simulink model "caracciolo"  (R2023b)
settings: Solver=FixedStepAuto  StartTime=0.0  StopTime=50  FixedStep=0.05  RelTol=1e-3
values from neighbouring files (symbols this model uses):
  a = 0.8    [init.m]
  b = 0.8    [init.m]
  d0 = 0.5    [init.m]
  fr = 0.005    [init.m]
  g = -9.8    [init.m]
  m = 550    [init.m]
  M = diag([m; m; I])    [init.m]
  M_inv = inv(M)    [init.m]
  mu = 0.9    [init.m]
  r = 0.3    [init.m]
  state0 = [0; 0; 0.2]    [init.m]
  tau_max = 3.88*2    (= 7.76)    [init.m]
  tau_min = -tau_max    (= -7.76)    [init.m]
libraries: simulink x1
settings Model: Creator=agisi2  LastModifiedBy=agisi2

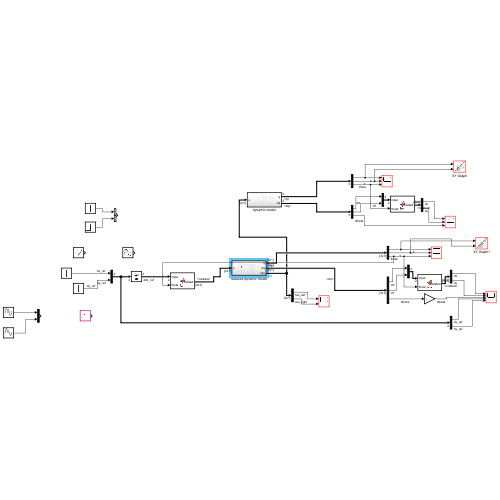
[thumbnail: Simulink's stored preview of the top-level diagram]
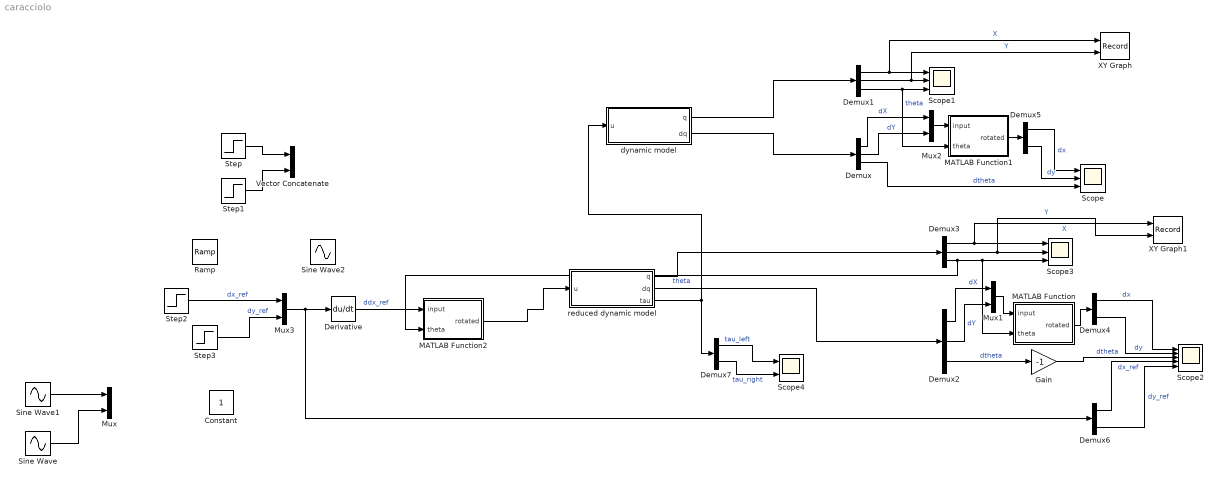
== system caracciolo ==
  Constant : Constant
  Demux{,1..3} (4 alike) : Demux  Outputs=3
  Demux{4..7} (4 alike) : Demux  Outputs=2
  Derivative : Derivative
  Gain : Gain  Gain=-1
  MATLAB Function : MATLAB Function  TreatAsAtomicUnit=on
  MATLAB Function1 : MATLAB Function  TreatAsAtomicUnit=on
  MATLAB Function2 : MATLAB Function  TreatAsAtomicUnit=on
  Mux{,1..3} (4 alike) : Mux  Inputs=2
  Ramp : simulink/Sources/Ramp  slope=1  start=1  InitialOutput=0
  Scope : Scope  NumInputPorts=3
  Scope1 : Scope  NumInputPorts=3
  Scope2 : Scope  NumInputPorts=5
  Scope3 : Scope  NumInputPorts=3
  Scope4 : Scope  NumInputPorts=2
  Sine Wave : Sin  SampleTime=0
  Sine Wave1 : Sin  SampleTime=0
  Sine Wave2 : Sin  SampleTime=0
  Step : Step  After=-2  SampleTime=0
  Step1 : Step  SampleTime=0
  Step2 : Step  Time=0.1  SampleTime=0
  Step3 : Step  Time=0.1  After=0  SampleTime=0
  Vector Concatenate : Concatenate
  XY Graph : Record  FileSettingsInternal="{\"entries\":[{\"content\":{\"excelSettings\":{\"content\":{},\"type\":\"Streamout.ExcelSettings\"}},\"type\":\"Streamout.FileSettingStorage\",\"uuid\":\"\"}],\"packageUris\":[\"http:\\/\\/schema.mathworks.com\\/mf0\\/streamout_blocks\\/R2020a\"],\"version\":\"1.0\"}"  Layout=[2 1]  SignalsInternal="{\"entries\":[{\"content\":{\"signals\":[{\"content\":{\"blockPath\":[],\"dimensions\":[1],\"domain\":\"\",\"lineColor\":\"#a2142f\",\"plots\":[1],\"port\":1,\"sid\":[\"\"],\"signalID\":5305,\"signalName\":\"X\"},\"type\":\"RecordBlkView.Signal\",\"uuid\":\"\"},{\"content\":{\"blockPath\":[],\"dimensions\":[1],\"domain\":\"\",\"lineColor\":\"#139fff\",\"plots\":[1],\"port\":2,\"sid\":[\"\"],\"signalID\":5309,\"signalName\":\"Y\"},\"type\":\"RecordBlkView.Signal\",\"uuid\":\"\"}]},\"type\":\"RecordBlkView.InputSignals\",\"uuid\":\"\"}],\"packageUris\":[\"http:\\/\\/schema.mathworks.com\\/mf0\\/streamout_blocks\\/R2020a\"],\"version\":\"1.0\"}"  VisualizationBindings="{\"xyplotplugin\":{\"info\":[{\"series\":[{\"bindingParametersList\":[{\"parameter\":\"X-Axis\",\"signalID\":5305,\"signalName\":\"X\"},{\"parameter\":\"Y-Axis\",\"signalID\":5309,\"signalName\":\"Y\"}],\"seriesID\":39005}],\"subplotID\":1},{\"series\":[],\"subplotID\":2}]}}"  CompatibilityTag=XY
  XY Graph1 : Record  FileSettingsInternal="{\"entries\":[{\"content\":{\"excelSettings\":{\"content\":{},\"type\":\"Streamout.ExcelSettings\"}},\"type\":\"Streamout.FileSettingStorage\",\"uuid\":\"\"}],\"packageUris\":[\"http:\\/\\/schema.mathworks.com\\/mf0\\/streamout_blocks\\/R2020a\"],\"version\":\"1.0\"}"  Layout=[1 1]  SignalsInternal="{\"entries\":[{\"content\":{\"signals\":[{\"content\":{\"blockPath\":[],\"dimensions\":[1,1],\"domain\":\"\",\"lineColor\":\"#a2142f\",\"plots\":[1],\"port\":1,\"sid\":[\"\"],\"signalID\":5313,\"signalName\":\"X\"},\"type\":\"RecordBlkView.Signal\",\"uuid\":\"\"},{\"content\":{\"blockPath\":[],\"dimensions\":[1,1],\"domain\":\"\",\"lineColor\":\"#139fff\",\"plots\":[1],\"port\":2,\"sid\":[\"\"],\"signalID\":5317,\"signalName\":\"Y\"},\"type\":\"RecordBlkView.Signal\",\"uuid\":\"\"}]},\"type\":\"RecordBlkView.InputSignals\",\"uuid\":\"\"}],\"packageUris\":[\"http:\\/\\/schema.mathworks.com\\/mf0\\/streamout_blocks\\/R2020a\"],\"version\":\"1.0\"}"  VisualizationBindings="{\"xyplotplugin\":{\"info\":[{\"series\":[{\"bindingParametersList\":[{\"parameter\":\"X-Axis\",\"signalID\":5313,\"signalName\":\"X\"},{\"parameter\":\"Y-Axis\",\"signalID\":5317,\"signalName\":\"Y\"}],\"seriesID\":47435}],\"subplotID\":1}]}}"  CompatibilityTag=XY
  dynamic model : Subsystem
  reduced dynamic model : Subsystem
  wires:
  dynamic model/2(dq) -> Demux/1
  dynamic model/1(q) -> Demux1/1
  Demux1/1 -> XY Graph/1, Scope1/1  "X"
  Demux1/2 -> XY Graph/2, Scope1/2  "Y"
  Demux1/3 -> MATLAB Function1/2(theta), Scope1/3  "theta"
  Demux/1 -> Mux2/1  "dX"
  Demux/2 -> Mux2/2  "dY"
  Demux/3 -> Scope/3  "dtheta"
  reduced dynamic model/2(dq) -> Demux2/1
  Demux2/3 -> Gain/1  "dtheta"
  Demux3/1 -> XY Graph1/1, Scope3/1  "X"
  reduced dynamic model/1(q) -> Demux3/1
  Demux3/2 -> XY Graph1/2, Scope3/2  "Y"
  Sine Wave/1 -> Mux/2
  Sine Wave1/1 -> Mux/1
  Step/1 -> Vector Concatenate/1
  Step1/1 -> Vector Concatenate/2
  Demux3/3 -> MATLAB Function2/2(theta), MATLAB Function/2(theta), Scope3/3  "theta"
  Mux1/1 -> MATLAB Function/1(input)
  Demux2/2 -> Mux1/2  "dY"
  Demux2/1 -> Mux1/1  "dX"
  MATLAB Function/1(rotated) -> Demux4/1
  Demux4/1 -> Scope2/1  "dx"
  Demux4/2 -> Scope2/2  "dy"
  Mux2/1 -> MATLAB Function1/1(input)
  MATLAB Function1/1(rotated) -> Demux5/1
  Demux5/1 -> Scope/1  "dx"
  Demux5/2 -> Scope/2  "dy"
  Step3/1 -> Mux3/2  "dy_ref"
  MATLAB Function2/1(rotated) -> reduced dynamic model/1(u)
  Mux3/1 -> Demux6/1, Derivative/1
  Demux6/1 -> Scope2/4  "dx_ref"
  Demux6/2 -> Scope2/5  "dy_ref"
  Step2/1 -> Mux3/1  "dx_ref"
  Derivative/1 -> MATLAB Function2/1(input)  "ddx_ref"
  Gain/1 -> Scope2/3  "dtheta"
  Demux7/1 -> Scope4/1  "tau_left"
  Demux7/2 -> Scope4/2  "tau_right"
  reduced dynamic model/3(tau) -> Demux7/1, dynamic model/1(u)

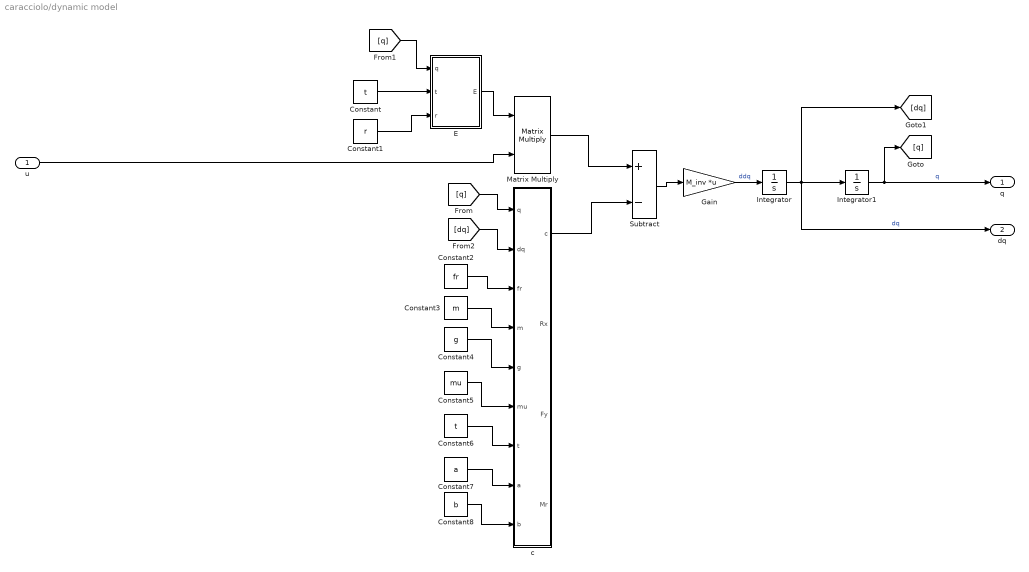
== system caracciolo/dynamic model ==
  u : Inport
  Constant : Constant  Value=t
  Constant1 : Constant  Value=r
  Constant2 : Constant  Value=fr
  Constant3 : Constant  Value=m
  Constant4 : Constant  Value=g
  Constant5 : Constant  Value=mu
  Constant6 : Constant  Value=t
  Constant7 : Constant  Value=a
  Constant8 : Constant  Value=b
  E : MATLAB Function  TreatAsAtomicUnit=on
  Gain : Gain  Gain=M_inv  Multiplication=Matrix(K*u) (u vector)
  Integrator : Integrator
  Integrator1 : Integrator  InitialCondition=state0
  Matrix Multiply : Product  Multiplication=Matrix(*)
  Subtract : Sum  Inputs=+-
  c : MATLAB Function  TreatAsAtomicUnit=on
  q : Outport
  dq : Outport  Port=2
  wires:
  E/1(E) -> Matrix Multiply/1
  u/1 -> Matrix Multiply/2
  Matrix Multiply/1 -> Subtract/1
  c/1(c) -> Subtract/2
  Subtract/1 -> Gain/1
  Gain/1 -> Integrator/1  "ddq"
  Integrator/1 -> dq/1, [dq], Integrator1/1  "dq"
  Integrator1/1 -> q/1, [q]  "q"
  [q] -> c/1(q)
  [q] -> E/1(q)
  [dq] -> c/2(dq)
  Constant/1 -> E/2(t)
  Constant1/1 -> E/3(r)
  Constant2/1 -> c/3(fr)
  Constant3/1 -> c/4(m)
  Constant4/1 -> c/5(g)
  Constant5/1 -> c/6(mu)
  Constant6/1 -> c/7(t)
  Constant7/1 -> c/8(a)
  Constant8/1 -> c/9(b)

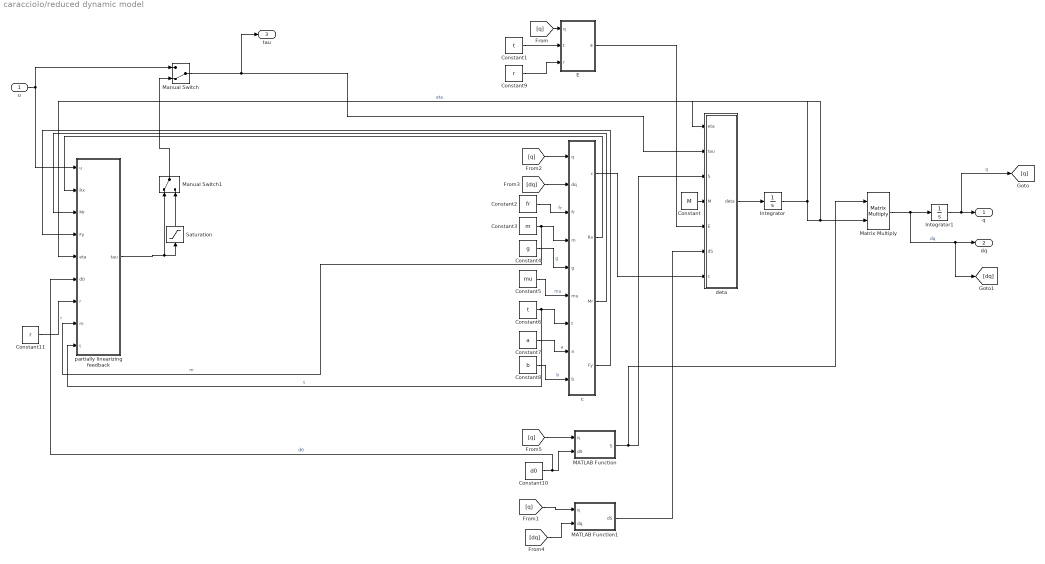
== system caracciolo/reduced dynamic model ==
  u : Inport
  Constant : Constant  Value=M
  Constant1 : Constant  Value=t
  Constant10 : Constant  Value=d0
  Constant11 : Constant  Value=r
  Constant2 : Constant  Value=fr
  Constant3 : Constant  Value=m
  Constant4 : Constant  Value=g
  Constant5 : Constant  Value=mu
  Constant6 : Constant  Value=t
  Constant7 : Constant  Value=a
  Constant8 : Constant  Value=b
  Constant9 : Constant  Value=r
  E : MATLAB Function  TreatAsAtomicUnit=on
  Integrator : Integrator
  Integrator1 : Integrator  InitialCondition=state0
  MATLAB Function : MATLAB Function  TreatAsAtomicUnit=on
  MATLAB Function1 : MATLAB Function  TreatAsAtomicUnit=on
  Manual Switch : ManualSwitch  CurrentSetting=0
  Manual Switch1 : ManualSwitch
  Matrix Multiply : Product  Multiplication=Matrix(*)
  Saturation : Saturate  UpperLimit=tau_max  LowerLimit=tau_min
  c : MATLAB Function  TreatAsAtomicUnit=on
  deta : MATLAB Function  TreatAsAtomicUnit=on
  partially linearizing feedback : MATLAB Function  TreatAsAtomicUnit=on
  q : Outport
  dq : Outport  Port=2
  tau : Outport  Port=3
  wires:
  Constant8/1 -> c/9(b)  "b"
  c/1(c) -> deta/7(c)
  Constant6/1 -> c/7(t), partially linearizing feedback/9(t)  "t"
  Constant4/1 -> c/5(g)  "g"
  Constant3/1 -> c/4(m), partially linearizing feedback/8(m)  "m"
  Constant7/1 -> c/8(a)  "a"
  Constant5/1 -> c/6(mu)  "mu"
  Constant2/1 -> c/3(fr)  "fr"
  Constant1/1 -> E/2(t)
  E/1(E) -> deta/5(E)
  Constant9/1 -> E/3(r)
  MATLAB Function/1(S) -> Matrix Multiply/1, deta/3(S)
  deta/1(deta) -> Integrator/1
  Integrator/1 -> partially linearizing feedback/5(eta), Matrix Multiply/2, deta/1(eta)  "eta"
  u/1 -> Manual Switch/1, partially linearizing feedback/1(u)
  Constant/1 -> deta/4(M)
  Matrix Multiply/1 -> [dq], dq/1, Integrator1/1  "dq"
  Integrator1/1 -> [q], q/1  "q"
  [q] -> MATLAB Function/1(q)
  [q] -> c/1(q)
  [dq] -> c/2(dq)
  [q] -> E/1(q)
  [q] -> MATLAB Function1/1(q)
  [dq] -> MATLAB Function1/2(dq)
  MATLAB Function1/1(dS) -> deta/6(dS)
  c/2(Rx) -> partially linearizing feedback/2(Rx)
  c/3(Mr) -> partially linearizing feedback/3(Mr)
  c/4(Fy) -> partially linearizing feedback/4(Fy)
  Constant10/1 -> partially linearizing feedback/6(d0), MATLAB Function/2(d0)  "d0"
  Constant11/1 -> partially linearizing feedback/7(r)  "r"
  partially linearizing feedback/1(tau) -> Saturation/1, Manual Switch1/1
  Manual Switch/1 -> tau/1, deta/2(tau)
  Manual Switch1/1 -> Manual Switch/2
  Saturation/1 -> Manual Switch1/2

== matlab function caracciolo/MATLAB Function ==
  data: input input; rotated output; theta input
function rotated = fcn(input, theta)
theta = -theta;
R = [cos(theta), -sin(theta); sin(theta), cos(theta)];
rotated = R * input;

== matlab function caracciolo/MATLAB Function1 ==
  data: input input; rotated output; theta input
function rotated = fcn(input, theta)

theta = -theta;
R = [cos(theta), -sin(theta); sin(theta), cos(theta)];
rotated = R * input;

== matlab function caracciolo/reduced dynamic model/partially linearizing feedback ==
  data: u input; tau output size=[2 1]; Rx input; Mr input; Fy input; eta input; d0 input; r input; m input; t input
function tau = fcn(u, Rx, Mr, Fy, eta, d0, r, m, t)

eta1 = eta(1);
eta2 = eta(2);
u1 = u(1);
u2 = u(2);

tau1 = (r/2) * (m*u1 + (m / d0)*eta2^2 + Rx) - (r*d0 / (2*t)) * ( (m+(1/d0^2)) * u2 - (m / d0) * eta1 * eta2 + Fy - (Mr / d0) );
tau2 = (r / 2) * (m*u1 + (m / d0)*eta2^2 + Rx) + (r*d0 / (2*t)) * ( (m + (1 / d0^2))*u2 - (m / d0) * eta1 * eta2 + Fy - (Mr / d0) );

tau = [tau1; tau2];

== matlab function caracciolo/MATLAB Function2 ==
  data: input input; rotated output; theta input
function rotated = fcn(input, theta)
theta = theta;
R = [cos(theta), -sin(theta); sin(theta), cos(theta)];
rotated = R * input;

== matlab function caracciolo/dynamic model/E ==
  data: q input; E output; t input; r input
function E = fcn(q, t, r)

theta = q(3);

E = [
    cos(theta) / r, cos(theta) / r;
    sin(theta) / r, sin(theta) / r;
    t / r, -t / r
];

== matlab function caracciolo/dynamic model/c ==
  data: q input; c output; dq input; fr input; m input; g input; mu input; t input; a input; b input; Rx output; Fy output; Mr output
function [c, Rx, Fy, Mr] = fcn(q, dq, fr, m, g, mu, t, a, b)

theta = q(3);
dX = dq(1);
dY = dq(2);
dtheta = dq(3);

dx = dX * cos(theta) - dY * sin(theta);
dy = dX * sin(theta) + dY * cos(theta);

dx1 = dx - t*dtheta;
dx2 = dx + t * dtheta;
dy1 = dy + a * dtheta;
dy3 = dy - b * dtheta;

Rx = fr * (m*g / 2) * (sign(dx1) + sign(dx2));
Fy = mu * (m*g / (a + b)) * (b * sign(dy1) + a * sign(dy3));
Mr = mu * (a*b*m*g / (a + b)) * (sign(dy1) - sign(dy3)) + fr*(t*m*g / 2) * (sign(dx2) - sign(dx1));

c1 = Rx * cos(theta) - Fy * sin(theta);
c2 = Rx * sin(theta) + Fy * cos(theta);
c3 = Mr;

c = [c1; c2; c3];

== matlab function caracciolo/reduced dynamic model/c ==
  data: q input; c output; dq input; fr input; m input; g input; mu input; t input; a input; b input; Rx output; Mr output; Fy output
function [c, Rx, Mr, Fy] = fcn(q, dq, fr, m, g, mu, t, a, b)
c = zeros(3, 1);

theta = q(3);
dX = dq(1);
dY = dq(2);
dtheta = dq(3);

dx = dX * cos(theta) - dY * sin(theta);
dy = dX * sin(theta) + dY * cos(theta);

dx1 = dx - t*dtheta;
dx2 = dx + t * dtheta;
dy1 = dy + a * dtheta;
dy3 = dy - b * dtheta;

Rx = fr * (m*g / 2) * (sign(dx1) + sign(dx2));
Fy = mu * (m*g / (a + b)) * (b * sign(dy1) + a * sign(dy3));
Mr = mu * (a*b*m*g / (a + b)) * (sign(dy1) - sign(dy3)) + fr*(t*m*g / 2) * (sign(dx2) - sign(dx1));

c1 = Rx * cos(theta) - Fy * sin(theta);
c2 = Rx * sin(theta) + Fy * cos(theta);
c3 = Mr;

c = [c1; c2; c3];

== matlab function caracciolo/reduced dynamic model/E ==
  data: q input; E output size=[3 2]; t input; r input
function E = fcn(q, t, r)
theta = q(3);

E = [
    cos(theta) / r, cos(theta) / r;
    sin(theta) / r, sin(theta) / r;
    t / r, -t / r
];

== matlab function caracciolo/reduced dynamic model/MATLAB Function ==
  data: q input; S output size=[3 2]; d0 input
function S = fcn(q, d0)

theta = q(3);
S = [cos(theta) -sin(theta); 
    sin(theta) cos(theta); 
    0 -1/d0];

== matlab function caracciolo/reduced dynamic model/deta ==
  data: eta input; deta output size=[2 1]; tau input; S input; M input; E input; dS input; c input
function deta = fcn(eta, tau, S, M, E, dS, c)

z = M*dS*eta;
deta = inv(S' * M * S) * S' * (E * tau - z - c);

== matlab function caracciolo/reduced dynamic model/MATLAB Function1 ==
  data: q input; dS output; dq input
function dS = fcn(q, dq)

theta = q(3);
dtheta = dq(3);

dS = [
    -sin(theta) * dtheta, -cos(theta)*dtheta; 
    cos(theta)*dtheta, -sin(theta)*dtheta; 
    0, 0
    ];
